simulink model "DFIG_and_Big_Generator"  (R2023a)
settings: Solver=ode45  StartTime=0.0  StopTime=10  RelTol=1e-2  EnableMultiTasking=on
PreLoadFcn:
  | assignin('base','Ts',[2e-6])
undefined symbols (not defined in the file): D1, Delta, DiscIntNeverNeededParam, find_system, Ion, level, Lithium, Ts
libraries: powerlib_extras x83, spsThreePhaseVIMeasurementLib x16, spsThreePhaseBreakerLib x16, simulink_extras x12, spsThreePhaseTransformerTwoWindingsLib x8, spsPLL3phLib x5, spsPowerPLLDrivenPositiveSequenceLib x5, spsUniversalBridgeLib x5, spsThreePhaseSeriesRLCLoadLib x5, spsThreePhaseSeriesRLCBranchLib x4, spsGroundLib x3, spsFundamentalPLLDrivenLib x2
(part 1 of 6)
settings Model: SimulationMode=accelerator  ExtModeTrigDuration=100  Creator=Administrator  LastModifiedBy=e36530cn
settings SolverCC: AlgebraicLoopSolver=TrustRegion
settings DataIOCC: LimitDataPoints=on  SaveFinalState=on  SaveFormat=Array  SignalLoggingSaveFormat=ModelDataLogs  SaveOutput=off  SaveState=on  ReturnWorkspaceOutputs=off  StateSaveName=tmp_raccel_xout
settings OptimizationCC: ExpressionDepthLimit=2147483647  EfficientMapNaN2IntZero=off  LifeSpan=inf
settings DebuggingCC: UnderspecifiedInitializationDetection=Classic  MergeDetectMultiDrivingBlocksExec=none  SolverPrmCheckMsg=warning  FcnCallInpInsideContextMsg=warning  UnconnectedInputMsg=warning  UnconnectedOutputMsg=warning  UnconnectedLineMsg=warning  StateNameClashWarn=warning  SFUnexpectedBacktrackingDiag=warning  SFNoUnconditionalDefaultTransitionDiag=warning  SFExecutionAtInitializationDiag=none  ArithmeticOperatorsInVariantConditions=warning
settings HardwareCC: ProdBitPerPointer=32  ProdBitPerSizeT=32  ProdBitPerPtrDiffT=32  ProdLargestAtomicFloat=None  ProdIntDivRoundTo=Undefined  ProdEndianess=Unspecified  ProdWordSize=32  ProdHWDeviceType=32-bit Generic  TargetBitPerPointer=64  TargetBitPerSizeT=64  TargetBitPerPtrDiffT=64  TargetLongLongMode=on  TargetIntDivRoundTo=Zero  TargetEndianess=LittleEndian  TargetWordSize=64  TargetHWDeviceType=MATLAB Host  ProdEqTarget=off
settings ModelReferenceCC: EnableRefExpFcnMdlSchedulingChecks=on  PropagateSignalLabelsOutOfModel=off
settings SFSimCC: SimUseLocalCustomCode=off  CustomCodeUndefinedFunction=UseInterfaceOnly
settings RTWCC: SystemTargetFile=raccel.tlc  TemplateMakefile=raccel_default_tmf  RTWVerbose=off  RTWUseLocalCustomCode=off  RTWUseSimCustomCode=on
settings CodeAppCC: GenerateComments=off  MaxIdLength=128  SimulinkBlockComments=off
settings RaccelTargetCC: ParMdlRefBuildCompliant=off  OptimizeReductions=off  ENABLE_SLEXEC_SSBRIDGE=0  RTWCAPISignals=off  RTWCAPIParams=off  RTWCAPIRootIO=off
settings ConfigComp: CovMetricSettings=dw  CovSaveCumulativeToWorkspaceVar=on  CovSaveSingleToWorkspaceVar=on  CovExternalEMLEnable=off
settings SimscapeCC: SimscapeNormalizeSystem=off

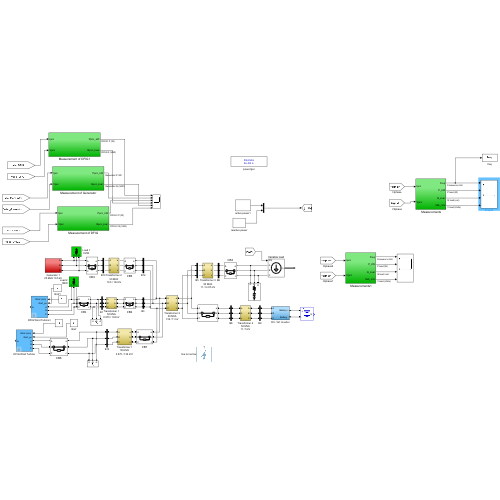
[thumbnail: Simulink's stored preview of the top-level diagram]
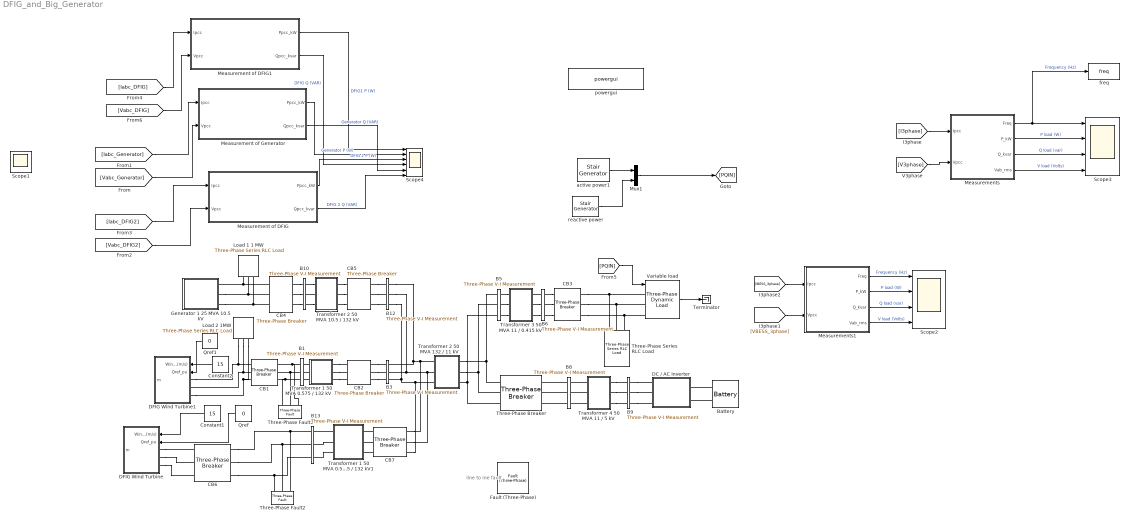
== system DFIG_and_Big_Generator ==
  note: line to ine fault
  " Measurements" : Subsystem
  " Measurements1" : Subsystem
  "B1 " : spsThreePhaseVIMeasurementLib/Three-Phase V-I Measurement  VoltageMeasurement=phase-to-ground  SetLabelV=on  LabelV=Vabc_DFIG  Vpu=off  VpuLL=off  CurrentMeasurement=yes  SetLabelI=on  LabelI=Iabc_DFIG  Ipu=off  Pbase=100e6  Vbase=735e3  OutputType=Complex  PhasorSimulation=off  PSBequivalent=0
  B10 : spsThreePhaseVIMeasurementLib/Three-Phase V-I Measurement  VoltageMeasurement=phase-to-ground  SetLabelV=on  LabelV=Vabc_Generator  Vpu=off  VpuLL=off  CurrentMeasurement=yes  SetLabelI=on  LabelI=Iabc_Generator  Ipu=off  Pbase=100e6  Vbase=735e3  OutputType=Complex  PhasorSimulation=off  PSBequivalent=0
  B12 : spsThreePhaseVIMeasurementLib/Three-Phase V-I Measurement  VoltageMeasurement=no  SetLabelV=on  LabelV=Vabc_B3  Vpu=off  VpuLL=off  CurrentMeasurement=no  SetLabelI=on  LabelI=Iabc_B2  Ipu=on  Pbase=100e6  Vbase=735e3  OutputType=Complex  PhasorSimulation=off  PSBequivalent=0
  B13 : spsThreePhaseVIMeasurementLib/Three-Phase V-I Measurement  VoltageMeasurement=phase-to-ground  SetLabelV=on  LabelV=Vabc_DFIG2  Vpu=off  VpuLL=off  CurrentMeasurement=yes  SetLabelI=on  LabelI=Iabc_DFIG2  Ipu=off  Pbase=100e6  Vbase=735e3  OutputType=Complex  PhasorSimulation=off  PSBequivalent=0
  "B3 " : spsThreePhaseVIMeasurementLib/Three-Phase V-I Measurement  VoltageMeasurement=no  SetLabelV=on  LabelV=Vabc_B3  Vpu=off  VpuLL=off  CurrentMeasurement=no  SetLabelI=on  LabelI=Iabc_B2  Ipu=on  Pbase=100e6  Vbase=735e3  OutputType=Complex  PhasorSimulation=off  PSBequivalent=0
  B5 : spsThreePhaseVIMeasurementLib/Three-Phase V-I Measurement  VoltageMeasurement=no  SetLabelV=on  LabelV=Vabc_B3  Vpu=off  VpuLL=off  CurrentMeasurement=no  SetLabelI=on  LabelI=Iabc_B2  Ipu=on  Pbase=100e6  Vbase=735e3  OutputType=Complex  PhasorSimulation=off  PSBequivalent=0
  B6 : spsThreePhaseVIMeasurementLib/Three-Phase V-I Measurement  VoltageMeasurement=phase-to-ground  SetLabelV=on  LabelV=V3phase  Vpu=off  VpuLL=off  CurrentMeasurement=yes  SetLabelI=on  LabelI=I3phase  Ipu=off  Pbase=100e6  Vbase=735e3  OutputType=Complex  PhasorSimulation=off  PSBequivalent=0
  B8 : spsThreePhaseVIMeasurementLib/Three-Phase V-I Measurement  VoltageMeasurement=no  SetLabelV=on  LabelV=Vabc_B3  Vpu=off  VpuLL=off  CurrentMeasurement=no  SetLabelI=on  LabelI=Iabc_B2  Ipu=on  Pbase=100e6  Vbase=735e3  OutputType=Complex  PhasorSimulation=off  PSBequivalent=0
  B9 : spsThreePhaseVIMeasurementLib/Three-Phase V-I Measurement  VoltageMeasurement=phase-to-ground  SetLabelV=on  LabelV=VBESS_3phase  Vpu=off  VpuLL=off  CurrentMeasurement=yes  SetLabelI=on  LabelI=IBESS_3phase  Ipu=off  Pbase=100e6  Vbase=735e3  OutputType=Complex  PhasorSimulation=off  PSBequivalent=0
  Battery : spsBatteryLib/Battery  BatType=Lithium-Ion  ShowTempParam=off  ThermalPreset=no  ShowAgeParam=off  NomV=5000  NomQ=13500  SOC=100  Batt_Tr=30  PresetModel=on  MaxQ=13500  MinV=3750  FullV=5819.9357  Dis_rate=5869.5652  R=0.0037037  Normal_OP=12208.6957  expZone="[5401.9293      663.26087]"  current=[2700 5400]  Units=Ampere-hour  Tci=20  NomT=25  T2=0  MaxQ2=2.208  FullV2=3.45  Normal_OP2=2.8  expZone2="[3.22        0.23]"  Rca=0.6  ti=1000  Dp=0  Neq0=0  Tsim=1e6  Ta1=25  Qeol=5.4*0.9  Reol=0.013333*1.2  Char_age=[2.3478, 3]  Dis_age=[2.3478, 10]  N1=1500  N2=10500  N3=1000  N4=1400  Ta2=45  N5=950
      settings: LibrarySourceBlock=electricdrivelib/Extra Sources/Battery
  CB{1..4} (4 alike) : spsThreePhaseBreakerLib/Three-Phase Breaker  InitialState=closed  SwitchA=off  SwitchB=off  SwitchC=off  SwitchTimes=[10]  External=off  BreakerResistance=1e-4  SnubberResistance=1e6  SnubberCapacitance=inf  Measurements=None
  CB5 : spsThreePhaseBreakerLib/Three-Phase Breaker  InitialState=closed  SwitchA=off  SwitchB=off  SwitchC=off  SwitchTimes=[1.360]  External=off  BreakerResistance=1e-4  SnubberResistance=1e6  SnubberCapacitance=inf  Measurements=None
  CB6 : spsThreePhaseBreakerLib/Three-Phase Breaker  InitialState=closed  SwitchA=off  SwitchB=off  SwitchC=off  SwitchTimes=[5,5.5]  External=off  BreakerResistance=1e-4  SnubberResistance=1e6  SnubberCapacitance=inf  Measurements=None
  CB7 : spsThreePhaseBreakerLib/Three-Phase Breaker  InitialState=closed  SwitchA=on  SwitchB=on  SwitchC=on  SwitchTimes=[5]  External=off  BreakerResistance=1e-4  SnubberResistance=1e6  SnubberCapacitance=inf  Measurements=None
  Constant1 : Constant  Value=15
  Constant2 : Constant  Value=15
  DC / AC Inverter : Subsystem
  DFIG Wind Turbine : Subsystem  LoadFcn=%find_system(gcs,'FollowLinks', 'on', 'LookUnderMasks', 'all');  mask(DFIG Wind Turbine){Nb_wt=8, ShowParameters=Turbine data for 1 wind turbine, nom=[1.5e6/.9 575 1975 50], sta=[ 0.023 0.18], rot=[ 0.016 0.16], Lm=2.9, mec=[0.685 0.01 3], init=[ -0.2,0   0,0,0   0,0,0 ], Imax_grid_conv=0.8, RL_grid=[ 0.3 0.003], Vdc_nom=1150, C_DClink1=10000e-6, C_var_filter1=120e3, Pmec1=1.5e6, wind_speed_CpMax=11, wind0=11, DisplayTurbChar=off, H_WT=4.32, Ksh=1.11, D_mutual=1.5, w_wt0=1.2, torque0=0.83, Kdc=[8   400], Kgrid_side_cur_reg=[0.83 5], Kspeed=[3 0.6], Krotor_side_cur_reg=[0.6 8], Ki_QV=[0.05 20], Kp_pitch=[150], Kcompensation=[3 30], PWM_freq_grid=2700, PWM_freq_rotor=1620, pitch_max=27, pitch_rate=10}
      mask prompts: Nb_wt "Number of wind turbines:"; ShowParameters "Display:"; nom "Nom. power, L-L volt. and freq. [Pn (VA), Vs_nom (Vrms), Vr_nom (Vrms), fn (Hz)]:"; sta "Stator [ Rs,Lls ] (p.u.):"; rot "Rotor [ Rr',Llr' ] (p.u.):"; Lm "Magnetizing inductance Lm (p.u.):"; mec "Inertia constant, friction factor, and pairs of poles [ H(s)  F(p.u.)  p ]:"; init "Initial conditions [s  th  ias  ibs  ics  phaseas phasebs phasecs]:"; Imax_grid_conv "Grid-side converter maximum current (pu of generator nominal current):"; RL_grid "Grid-side coupling inductor [ L, R] (p.u.):"; Vdc_nom "Nominal DC bus voltage (V):"; C_DClink1 "DC bus capacitor (F):"; C_var_filter1 "Line filter capacitor (Q=50) (var):"; Pmec1 "Nominal mechanical output power (W):"; wind_speed_CpMax "Wind speed at nominal speed and at Cp max (must be between 6 m/s and 30 m/s) (m/s):"; wind0 "Initial wind speed (m/s):"; DisplayTurbChar "Display wind turbine power characteristics:"; H_WT "Wind turbine inertia constant H (s):"; Ksh "Shaft spring constant refer to high-speed shaft (pu of nominal mechanical torque/rad):"; D_mutual "Shaft mutual damping (pu of nominal mechanical torque/pu dw):"; w_wt0 "Turbine initial speed (pu of nominal speed):"; torque0 "Initial output torque (pu of nominal mechanical torque):"; Kdc "DC bus voltage regulator gains [Kp Ki]:"; Kgrid_side_cur_reg "Grid-side converter current regulator gains [Kp Ki]:"; Kspeed "Speed regulator gains [Kp Ki]:"; Krotor_side_cur_reg "Rotor-side converter current regulator gains [Kp Ki]:"; Ki_QV "Q and V regulator gains [Ki_var Ki_volt]:"; Kp_pitch "Pitch controller gain [Kp]:"; Kcompensation "Pitch compensation gains [Kp Ki]:"; PWM_freq_grid "Frequency of the grid-side PWM carrier (Hz):"; PWM_freq_rotor "Frequency of the rotor-side PWM carrier (Hz):"; pitch_max "Maximum pitch angle (deg):"; pitch_rate "Maximum rate of change of pitch angle (deg/s):"
      mask help: This block implements a model of a variable speed pitch controlled wind turbine using a doubly-fed induction generator (DFIG).
      mask init:
      | %Generator data
      | Pnom=nom(1)*Nb_wt;
      | Vnom=nom(2);
      | Vnom_r=nom(3);
      | Fnom=nom(4);
      | Rs=sta(1);
      | Lls=sta(2);
      | Rr=rot(1);
      | Llr=rot(2);
      | H=mec(1);
      | F=mec(2);
      | p=mec(3);
      | 
      | % Converters data
      | L_RL=RL_grid(1);
      | R_RL=RL_grid(2);
      | Q_filter=50;
      | C_DClink=C_DClink1*Nb_wt;
      | C_var_filter=C_var_filter1*Nb_wt;
      | 
      | % Controller data
      | Freq_filter=1000*10;   %Hz
      | Zeta_filter=0.707;
      | Mod_index_max_grid=1.1;   %Maximum value of modulation index for grid-side converter
      | Mod_index_max_rotor=2;   %Maximum value of modulation index for rotor-side converter
      | Lim_grid_side_cur_reg=1.1; %Limit for grid-side PI current regulator (pu)
      | Lim_rotor_side_cur_reg=0.1; %Limit for rotor-side PI current regulator (pu)
      | Min_var_reg=0.9; %Minimum output value for integral var regulator (pu)
      | Max_var_reg=1.1; %Maximum output value for integral var regulator (pu)
      | Max_speed_reg=1; %Maximum output value for PI speed regulator (pu)
      | Kp_dc=Kdc(1);
      | Ki_dc=Kdc(2);
      | Kp_grid_side_cur_reg=Kgrid_side_cur_reg(1);
      | Ki_grid_side_cur_reg=Kgrid_side_cur_reg(2);
      | Kp_speed=Kspeed(1);
      | Ki_speed=Kspeed(2);
      | Kp_compensation=Kcompensation(1);
      | Ki_compensation=Kcompensation(2);
      | Kp_rotor_side_cur_reg=Krotor_side_cur_reg(1);
      | Ki_rotor_side_cur_reg=Krotor_side_cur_reg(2);
      | Ki_var=Ki_QV(1);
      | Ki_volt=Ki_QV(2);
      | Iq_ref_limit_time_constant=0.3; %(s)
      | T_speed=5;      %s
      | Min_mag_flux=0.5;   %(pu)
      | Max_Idr_ref=0.9;    %(pu)
      | Speed_max=1.2;  %(pu)
      | Speed_min=0.7;  %(pu)
      | Pitch_time_constant=0.01;    %(s)
      | 
      | 
      | % Turbine data
      | Pmec=Pmec1*Nb_wt;
      | c1 = 0.6450;
      | c2 = 116;
      | c3 = .4;
      | c4 = 5;
      | c5 = 21;
      | c6 = .00912;  % Set Pmin in stall condition (does not vary with wind_speed_Pmax)
      | c7 = .08;
      | c8 = .035;
      | theta=0;
      | CpMax=.5;
      | lambda_CpMax=9.9495;
      | 
      | c1_c8=[c1 c2 c3 c4 c5 c6 c7 c8];
      |   
      | 
      | %   Cp = c1*(c6*lambda + (-c4 - c3*(2.5 + theta) + c2*(1/(lambda + ...
      | %   c7*(2.5 + theta)) - c8/(1 + (2.5 + theta)^3)))/exp(c5*(1/(lambda + ...
      | %   c7*(2.5 + theta)) - c8/(1 + (2.5 + theta)^3))))
      | 
      | 
      |         %%%%%%%%%%%%%%%%%%%%%%%%%%%%%%%%%%%%%%%%%%%%%%%%%%%%%%%%%%%%%%%%%%%%%%%%%%%
      |         % Operation at Cp max
      |         %%%%%%%%%%%%%%%%%%%%%%%%%%%%%%%%%%%%%%%%%%%%%%%%%%%%%%%%%%%%%%%%%%%%%%%%%%%
      |         
      |         rated_omegar=1.2;
      |         omegar = rated_omegar;
      |         
      |         % Enforce boundaries on wind speed
      |         % A warning could be displayed
      |         if wind_speed_CpMax < 6
      |             wind_speed_CpMax=6;
      |             disp('Warning: Wind speed at nominal speed and at Cp max has been set to 6 m/s')
      |         end
      |         if wind_speed_CpMax > 30
      |             wind_speed_CpMax=30;
      |             disp('Warning: Wind speed at nominal speed and at Cp max has been set to 30 m/s')
      |         end
      | 
      |         K1=lambda_CpMax/omegar*wind_speed_CpMax;
      |         
      |         % Calculation of K2 needed to get P equal to the requested value at
      |         % Cp max for the requested wind speed
      |         
      |         Prated=Pmec1*Nb_wt;
      |         P_rated_omegar_theta_zero=0.75;
      |         
      |         K2 = P_rated_omegar_theta_zero*Prated/(wind_speed_CpMax^3*CpMax);
      |         
      |         K1_K2=[K1 K2];
      |         
      |         %%%%%%%%%%%%%%%%%%%%%%%%%%%%%%%%%%%%%%%%%%%%%%%%%%%%%%%%%%%%%%%%%%%%%%%%%%%
      |         % End of calculation for operation at Cp max
      |         %%%%%%%%%%%%%%%%%%%%%%%%%%%%%%%%%%%%%%%%%%%%%%%%%%%%%%%%%%%%%%%%%%%%%%%%%%%
      |         
      | 
      | %%%%%%%%%%%%%%%%%%%%%%%%%%%%%%%%%%%%%%%%%%%%%%%%%%%%%%%%%%%%%%%%%%%%%%%%%%%
      | % Plot turbine characteristics
      | %%%%%%%%%%%%%%%%%%%%%%%%%%%%%%%%%%%%%%%%%%%%%%%%%%%%%%%%%%%%%%%%%%%%%%%%%%% 
      | 
      | DisplayTurbChar=get_param(gcb,'DisplayTurbChar');
      | if strcmp(DisplayTurbChar,'on')
      |     vect_theta = 0:2:30;
      |     
      |     vect_lambda = 1:0.2:30;
      |     
      |     clear Cp;
      |     
      |     for i=1:length(vect_theta)
      |      for j=1:length(vect_lambda)
      |                 Cp(i,j) = c1*(c6*vect_lambda(j) + (-c4 - c3*(2.5 + vect_theta(i)) + c2*(1/(vect_lambda(j) + ...
      |                 c7*(2.5 + vect_theta(i))) - c8/(1 + (2.5 + vect_theta(i))^3)))/exp(c5*(1/(vect_lambda(j) + ...
      |                 c7*(2.5 + vect_theta(i))) - c8/(1 + (2.5 + vect_theta(i))^3))));
      |      end
      |     end
      | 
      |     figure(1);
      |     clf;
      |     hold on;
      | 
      |     plot(vect_lambda, Cp);
      |     axis([0, 25, 0, .6]);
      |     title('Wind Turbine Cp Characteristic (pitch angle increases by step of 2 deg.)');
      |     ylabel('Cp');
      |     set(gca,'ytick',[0 .1 .2 .3 .4 .5 .6]);
      |     xlabel('Lambda');
      |     grid on;
      |     text(10.1,0.51,'Pitch angle 0 degree');
      | 
      |     hold off
      |     
      |     % Plot of the wind turbine mechanical power output (pu) lambda and Cp
      |     % characteristics against wind speed (m/s) for a range of theta.
      |     
      |     wind_speed_range = [1,.2,30];
      |     vect_wind_speed = 1:0.2:30;
      |     
      |     clear lambda;
      |     clear Cp;
      |     clear P;
      | 
      |     for i=1:length(vect_theta)
      |         for j=1:length(vect_wind_speed)
      |             lambda(i,j) = K1*omegar/vect_wind_speed(j);
      |             Cp(i,j) = c1*(c6*lambda(i,j) + (-c4 - c3*(2.5 + vect_theta(i)) + c2*(1/(lambda(i,j) + ...
      |             c7*(2.5 + vect_theta(i))) - c8/(1 + (2.5 + vect_theta(i))^3)))/exp(c5*(1/(lambda(i,j) + ...
      |             c7*(2.5 + vect_theta(i))) - c8/(1 + (2.5 + vect_theta(i))^3))));
      |             P(i,j) = K2/Prated*vect_wind_speed(j)^3*Cp(i,j);
      |         end
      |     end
      |     
      |     
      |     figure(2);
      |     clf;
      |     hold on
      |     
      |     subplot(3,1,1);
      |     plot(vect_wind_speed, P);
      |     axis([0, 35, 0, 1.5]);
      |     title('Wind Turbine Characteristics (w = 1.2 pu, pitch angle increases by step of 2 deg.)');
      |     ylabel('P (pu)');
      |     set(gca,'ytick',0:.5:4);
      |     grid on;
      |     
      |     subplot(3,1,2);
      |     plot(vect_wind_speed, lambda);
      |     axis([0, 35, 0, 20]);
      |     ylabel('Lambda');
      |     grid on;
      |     
      |     subplot(3,1,3)
      |     plot(vect_wind_speed, Cp);
      |     axis([0, 35, 0, .6]);
      |     xlabel('Wind Speed (m/s)');
      |     ylabel('Cp');
      |     set(gca,'ytick',[0 .1 .2 .3 .4 .5 .6]);
      |     grid on;
      | 
      |     hold off
      |     set_param(gcb,'DisplayTurbChar','off')
      |     
      | end
      mask TypeOptions ShowParameters: Generator data for 1 wind turbine | Converters data for 1 wind turbine | Turbine data for 1 wind turbine | Drive train data for 1 wind turbine | Control parameters for 1 wind turbine
      mask Callback ShowParameters:
      | BlockName=getfullname(gcb);
      | %
      | Param_Show=get_param(BlockName,'ShowParameters');
      | Param_DisplayTurbChar=get_param(BlockName,'DisplayTurbChar');
      | 
      | p_mask{3}='off';p_mask{4}='off';p_mask{5}='off';
      | p_mask{6}='off';p_mask{7}='off';p_mask{8}='off';p_mask{9}='off';
      | p_mask{10}='off';p_mask{11}='off';p_mask{12}='off';p_mask{13}='off';
      | p_mask{14}='off';p_mask{15}='off';p_mask{16}='off';p_mask{17}='off';
      | p_mask{18}='off';p_mask{19}='off';p_mask{20}='off';p_mask{21}='off';
      | p_mask{22}='off';p_mask{23}='off';p_mask{24}='off';p_mask{25}='off';
      | p_mask{26}='off';p_mask{27}='off';p_mask{28}='off';p_mask{29}='off';
      | p_mask{30}='off';p_mask{31}='off';p_mask{32}='off';p_mask{33}='off';
      | 
      | 
      | switch Param_Show
      | 	case 'Generator data for 1 wind turbine'
      | 		p_mask{3}='on';p_mask{4}='on';p_mask{5}='on'; p_mask{6}='on';
      |         p_mask{7}='on'; p_mask{8}='on';
      |     case 'Converters data for 1 wind turbine'
      | 		p_mask{9}='on';p_mask{10}='on';p_mask{11}='on';p_mask{12}='on';
      |         p_mask{13}='on';
      | 	case 'Turbine data for 1 wind turbine'
      |         p_mask{14}='on';p_mask{15}='on';p_mask{16}='on';p_mask{17}='on';
      |     case 'Drive train data for 1 wind turbine'
      |         p_mask{18}='on';p_mask{19}='on';p_mask{20}='on';p_mask{21}='on';
      |         p_mask{22}='on';
      |     case 'Control parameters for 1 wind turbine'
      |         p_mask{23}='on';p_mask{24}='on';p_mask{25}='on';
      |         p_mask{26}='on';p_mask{27}='on';p_mask{28}='on';p_mask{29}='on';
      |         p_mask{30}='on'; p_mask{31}='on';p_mask{32}='on'; p_mask{33}='on';
      | end
      | 
      | ParVisible={'on','on',p_mask{3},p_mask{4},p_mask{5},p_mask{6},p_mask{7},...
      |     p_mask{8},p_mask{9},p_mask{10},p_mask{11},p_mask{12},p_mask{13},...
      |     p_mask{14},p_mask{15},p_mask{16},p_mask{17},p_mask{18},p_mask{19},...
      |     p_mask{20},p_mask{21},p_mask{22},p_mask{23},p_mask{24},p_mask{25},...
      |     p_mask{26},p_mask{27},p_mask{28},p_mask{29},p_mask{30},p_mask{31},...
      |     p_mask{32},p_mask{33}};
      | %
      | set_param(BlockName,'MaskVisibilities',ParVisible);
      | set_param(BlockName,'DisplayTurbChar',Param_DisplayTurbChar);
  DFIG Wind Turbine1 : Subsystem  LoadFcn=%find_system(gcs,'FollowLinks', 'on', 'LookUnderMasks', 'all');  mask(DFIG Wind Turbine){Nb_wt=9, ShowParameters=Turbine data for 1 wind turbine, nom=[1.5e6/.9 575 1975 50], sta=[ 0.023 0.18], rot=[ 0.016 0.16], Lm=2.9, mec=[0.685 0.01 3], init=[ -0.2,0   0,0,0   0,0,0 ], Imax_grid_conv=0.8, RL_grid=[ 0.3 0.003], Vdc_nom=1150, C_DClink1=10000e-6, C_var_filter1=120e3, Pmec1=1.5e6, wind_speed_CpMax=11, wind0=11, DisplayTurbChar=off, H_WT=4.32, Ksh=1.11, D_mutual=1.5, w_wt0=1.2, torque0=0.83, Kdc=[8   400], Kgrid_side_cur_reg=[0.83 5], Kspeed=[3 0.6], Krotor_side_cur_reg=[0.6 8], Ki_QV=[0.05 20], Kp_pitch=[150], Kcompensation=[3 30], PWM_freq_grid=2700, PWM_freq_rotor=1620, pitch_max=27, pitch_rate=10}
      mask prompts: Nb_wt "Number of wind turbines:"; ShowParameters "Display:"; nom "Nom. power, L-L volt. and freq. [Pn (VA), Vs_nom (Vrms), Vr_nom (Vrms), fn (Hz)]:"; sta "Stator [ Rs,Lls ] (p.u.):"; rot "Rotor [ Rr',Llr' ] (p.u.):"; Lm "Magnetizing inductance Lm (p.u.):"; mec "Inertia constant, friction factor, and pairs of poles [ H(s)  F(p.u.)  p ]:"; init "Initial conditions [s  th  ias  ibs  ics  phaseas phasebs phasecs]:"; Imax_grid_conv "Grid-side converter maximum current (pu of generator nominal current):"; RL_grid "Grid-side coupling inductor [ L, R] (p.u.):"; Vdc_nom "Nominal DC bus voltage (V):"; C_DClink1 "DC bus capacitor (F):"; C_var_filter1 "Line filter capacitor (Q=50) (var):"; Pmec1 "Nominal mechanical output power (W):"; wind_speed_CpMax "Wind speed at nominal speed and at Cp max (must be between 6 m/s and 30 m/s) (m/s):"; wind0 "Initial wind speed (m/s):"; DisplayTurbChar "Display wind turbine power characteristics:"; H_WT "Wind turbine inertia constant H (s):"; Ksh "Shaft spring constant refer to high-speed shaft (pu of nominal mechanical torque/rad):"; D_mutual "Shaft mutual damping (pu of nominal mechanical torque/pu dw):"; w_wt0 "Turbine initial speed (pu of nominal speed):"; torque0 "Initial output torque (pu of nominal mechanical torque):"; Kdc "DC bus voltage regulator gains [Kp Ki]:"; Kgrid_side_cur_reg "Grid-side converter current regulator gains [Kp Ki]:"; Kspeed "Speed regulator gains [Kp Ki]:"; Krotor_side_cur_reg "Rotor-side converter current regulator gains [Kp Ki]:"; Ki_QV "Q and V regulator gains [Ki_var Ki_volt]:"; Kp_pitch "Pitch controller gain [Kp]:"; Kcompensation "Pitch compensation gains [Kp Ki]:"; PWM_freq_grid "Frequency of the grid-side PWM carrier (Hz):"; PWM_freq_rotor "Frequency of the rotor-side PWM carrier (Hz):"; pitch_max "Maximum pitch angle (deg):"; pitch_rate "Maximum rate of change of pitch angle (deg/s):"
      mask help: This block implements a model of a variable speed pitch controlled wind turbine using a doubly-fed induction generator (DFIG).
      mask init: same as DFIG_and_Big_Generator/DFIG Wind Turbine
      mask TypeOptions ShowParameters: Generator data for 1 wind turbine | Converters data for 1 wind turbine | Turbine data for 1 wind turbine | Drive train data for 1 wind turbine | Control parameters for 1 wind turbine
      mask Callback ShowParameters:
      | BlockName=getfullname(gcb);
      | %
      | Param_Show=get_param(BlockName,'ShowParameters');
      | Param_DisplayTurbChar=get_param(BlockName,'DisplayTurbChar');
      | 
      | p_mask{3}='off';p_mask{4}='off';p_mask{5}='off';
      | p_mask{6}='off';p_mask{7}='off';p_mask{8}='off';p_mask{9}='off';
      | p_mask{10}='off';p_mask{11}='off';p_mask{12}='off';p_mask{13}='off';
      | p_mask{14}='off';p_mask{15}='off';p_mask{16}='off';p_mask{17}='off';
      | p_mask{18}='off';p_mask{19}='off';p_mask{20}='off';p_mask{21}='off';
      | p_mask{22}='off';p_mask{23}='off';p_mask{24}='off';p_mask{25}='off';
      | p_mask{26}='off';p_mask{27}='off';p_mask{28}='off';p_mask{29}='off';
      | p_mask{30}='off';p_mask{31}='off';p_mask{32}='off';p_mask{33}='off';
      | 
      | 
      | switch Param_Show
      | 	case 'Generator data for 1 wind turbine'
      | 		p_mask{3}='on';p_mask{4}='on';p_mask{5}='on'; p_mask{6}='on';
      |         p_mask{7}='on'; p_mask{8}='on';
      |     case 'Converters data for 1 wind turbine'
      | 		p_mask{9}='on';p_mask{10}='on';p_mask{11}='on';p_mask{12}='on';
      |         p_mask{13}='on';
      | 	case 'Turbine data for 1 wind turbine'
      |         p_mask{14}='on';p_mask{15}='on';p_mask{16}='on';p_mask{17}='on';
      |     case 'Drive train data for 1 wind turbine'
      |         p_mask{18}='on';p_mask{19}='on';p_mask{20}='on';p_mask{21}='on';
      |         p_mask{22}='on';
      |     case 'Control parameters for 1 wind turbine'
      |         p_mask{23}='on';p_mask{24}='on';p_mask{25}='on';
      |         p_mask{26}='on';p_mask{27}='on';p_mask{28}='on';p_mask{29}='on';
      |         p_mask{30}='on'; p_mask{31}='on';p_mask{32}='on'; p_mask{33}='on';
      | end
      | 
      | ParVisible={'on','on',p_mask{3},p_mask{4},p_mask{5},p_mask{6},p_mask{7},...
      |     p_mask{8},p_mask{9},p_mask{10},p_mask{11},p_mask{12},p_mask{13},...
      |     p_mask{14},p_mask{15},p_mask{16},p_mask{17},p_mask{18},p_mask{19},...
      |     p_mask{20},p_mask{21},p_mask{22},p_mask{23},p_mask{24},p_mask{25},...
      |     p_mask{26},p_mask{27},p_mask{28},p_mask{29},p_mask{30},p_mask{31},...
      |     p_mask{32},p_mask{33}};
      | %
      | set_param(BlockName,'MaskVisibilities',ParVisible);
      | set_param(BlockName,'DisplayTurbChar',Param_DisplayTurbChar);
  Fault (Three-Phase) : ee_lib/Utilities/Fault (Three-Phase)  fault_type_option=0  R_pn_fault=1e-3 Ohm  R_ng_fault=1e-3 Ohm  exposemeasurement=ee.enum.exposemeasurement.hidden  enable_external_fault=ee.enum.external_fault.hidden  fault_threshold=0.5  fault_condition=1  fault_resettable=0  enable_temporal_fault=0  fault_start_time=1 s  fault_duration=0.1 s  G_parasitic=1e-6 1/Ohm
      settings: InternalSimscapePortConfiguration="{\"Bottom\":[],\"Left\":[{\"id\":\"N\",\"label\":\"~\",\"type\":\"foundation.electrical.three_phase\"}],\"Right\":[],\"Top\":[]}"
  Generator 1 25 MVA 10.5 kV : Subsystem
  Load 1 1 MW : spsThreePhaseSeriesRLCLoadLib/Three-Phase Series RLC Load  LConnTagsString=A|B|C  Configuration=Y (grounded)  NominalVoltage=10.5e3  Vabc=[1e3 1e3 1e3]  Vabcp=[1e3 1e3 1e3]  NominalFrequency=50  UnbalancedPower=off  ActivePower=1e6  InductivePower=0  CapacitivePower=0  Pabc=[10e3 9e3 11e3]  QLabc=[100 90 110]  QCabc=[100 90 110]  Pabcp=[10e3 9e3 11e3]  QLabcp=[100 90 110]  QCabcp=[100 90 110]  Measurements=None  LoadType=constant Z
  Load 2 1MW : spsThreePhaseSeriesRLCLoadLib/Three-Phase Series RLC Load  LConnTagsString=A|B|C  Configuration=Y (grounded)  NominalVoltage=575  Vabc=[1e3 1e3 1e3]  Vabcp=[1e3 1e3 1e3]  NominalFrequency=50  UnbalancedPower=off  ActivePower=1e6  InductivePower=0  CapacitivePower=0  Pabc=[10e3 9e3 11e3]  QLabc=[100 90 110]  QCabc=[100 90 110]  Pabcp=[10e3 9e3 11e3]  QLabcp=[100 90 110]  QCabcp=[100 90 110]  Measurements=None  LoadType=constant Z
  Measurement of DFIG : Subsystem
  Measurement of DFIG1 : Subsystem
  Measurement of Generator : Subsystem
  Mux1 : Mux  Inputs=2
  Qref : Constant  Value=0
  Qref1 : Constant  Value=0
  Scope2 : Scope  NumInputPorts=4
  Scope3 : Scope  NumInputPorts=4
  Scope4 : Scope  NumInputPorts=6
  Terminator : Terminator
  Three-Phase Series RLC Load : spsThreePhaseSeriesRLCLoadLib/Three-Phase Series RLC Load  LConnTagsString=A|B|C  Configuration=Y (grounded)  NominalVoltage=415  Vabc=[1e3 1e3 1e3]  Vabcp=[1e3 1e3 1e3]  NominalFrequency=50  UnbalancedPower=off  ActivePower=15E6  InductivePower=0  CapacitivePower=27E6  Pabc=[10e3 9e3 11e3]  QLabc=[100 90 110]  QCabc=[100 90 110]  Pabcp=[10e3 9e3 11e3]  QLabcp=[100 90 110]  QCabcp=[100 90 110]  Measurements=None  LoadType=constant Z
  Three-Phase Breaker : spsThreePhaseBreakerLib/Three-Phase Breaker  InitialState=closed  SwitchA=off  SwitchB=off  SwitchC=off  SwitchTimes="[1/60  5/60]"  External=off  BreakerResistance=0.01  SnubberResistance=1e6  SnubberCapacitance=inf  Measurements=None
  Three-Phase Fault1 : spsThreePhaseFaultLib/Three-Phase Fault  InitialStates=0  FaultA=on  FaultB=off  FaultC=off  GroundFault=off  SwitchTimes=[ 5]  External=off  SwitchStatus=NaN  FaultResistance=0.001  GroundResistance=0.01  SnubberResistance=1e6  SnubberCapacitance=inf  Measurements=None
  Three-Phase Fault2 : spsThreePhaseFaultLib/Three-Phase Fault  InitialStates=0  FaultA=off  FaultB=off  FaultC=off  GroundFault=off  SwitchTimes=[5]  External=off  SwitchStatus=NaN  FaultResistance=0.001  GroundResistance=0.01  SnubberResistance=1e6  SnubberCapacitance=inf  Measurements=None
  Transformer 1 50 MVA 0.575 / 132 kV : Subsystem
  Transformer 1 50 MVA 0.575 / 132 kV1 : Subsystem
  Transformer 2 50 MVA 10.5 / 132 kV : Subsystem
  Transformer 2 50 MVA 132 / 11 kV : Subsystem
  Transformer 3 50 MVA 11 / 0.415 kV : Subsystem
  Transformer 4 50 MVA 11 / 5 kV : Subsystem
  Variable load : spsThreePhaseDynamicLoadLib/Three-Phase Dynamic Load  NominalVoltage=[ 415 50 ]  ActiveReactivePowers=[15e6 0E6]  PositiveSequence=[1 0]  ExternalControl=on  NpNq=[1.3 2]  TimeConstants="[0  0  0  0]"  MinimumVoltage=0.7  Tfilter=1e-4  LoadFlowParameters=[4,0,0,0,0]
  active power1 : spsStairGeneratorLib/Stair Generator  t=[0]  e=[15E6]  Ts=0
  freq : ToWorkspace  VariableName=freq  SaveFormat=Structure With Time  SampleTime=-1
  powergui : sps_lib/powergui  Priority=1  SimulationMode=Discrete  SampleTime=Ts  frequency=60  Iterations=50  frequencyindice=0  Pbase=100e6  ErrMax=1e-4  UnitsV=kV  UnitsW=MW  buscounter=0  FunctionMessages=off  echomessages=off  EnableUseOfTLC=off  CurrentSourceSwitches=off  DisableSnubberDevices=off  DisableRonSwitches=off  DisableVfSwitches=off  DisplayEquations=off  AutomaticDiscreteSolvers=off  SolverType=Tustin  Interpol=off  ExternalGateDelay=off  methode=off  Ts=10  x0status=blocks  SPID=off  SwTol=0  HookPort=off  NonlinearTolerance=1e-4  nMaxIteration=100  ContinueOnMaxIteration=off  RestoreLinks=warning  ResistiveCurrentMeasurement=off  Frange=[0:2:500]  Ylog=off  Xlog=on  ShowGrid=off  save=off  variable=ZData  structure=psbbridges_str  ZoomFFT=off  StartTime=0.0  cycles=1  DisplayStyle=1  fundamental=50  FreqAxis=off  MaxFrequency=100  frequencyindicesteady=1  RmsSteady=2  display=off
  reactive power : spsStairGeneratorLib/Stair Generator  t=[0]  e=[0]  Ts=0
  Scope1 : Scope
  wires:
  [V3phase] -> " Measurements"/2(Vpcc)
  " Measurements"/1(Freq) -> freq/1, Scope3/1  "Frequency (Hz)"
  [I3phase] -> " Measurements"/1(Ipcc)
  " Measurements"/3(Q_kvar) -> Scope3/3  "Q load (var)"
  " Measurements"/2(P_kW) -> Scope3/2  "P load (W)"
  " Measurements"/4(Vab_rms) -> Scope3/4  "V load (Volts)"
  Measurement of DFIG/1(Ppcc_kW) -> Scope4/3  "DFIG 2 P (W)"
  Measurement of DFIG/2(Qpcc_kvar) -> Scope4/6  "DFIG 2 Q (VAR)"
  [Vabc_Generator] -> Measurement of Generator/2(Vpcc)
  [Iabc_Generator] -> Measurement of Generator/1(Ipcc)
  [Vabc_DFIG2] -> Measurement of DFIG/2(Vpcc)
  [Iabc_DFIG2] -> Measurement of DFIG/1(Ipcc)
  Qref/1 -> DFIG Wind Turbine/2(Qref_pu)
  Constant1/1 -> DFIG Wind Turbine/1("Wind (m/s) ")
  Qref1/1 -> DFIG Wind Turbine1/2(Qref_pu)
  Constant2/1 -> DFIG Wind Turbine1/1("Wind (m/s) ")
  [Iabc_DFIG] -> Measurement of DFIG1/1(Ipcc)
  [Vabc_DFIG] -> Measurement of DFIG1/2(Vpcc)
  Measurement of DFIG1/2(Qpcc_kvar) -> Scope4/4  "DFIG Q (VAR)"
  Measurement of DFIG1/1(Ppcc_kW) -> Scope4/1  "DFIG1 P (W)"
  Variable load/1 -> Terminator/1
  Mux1/1 -> [PQIN]
  reactive power/1 -> Mux1/2
  active power1/1 -> Mux1/1
  Measurement of Generator/1(Ppcc_kW) -> Scope4/2  "Generator P (W)"
  Measurement of Generator/2(Qpcc_kvar) -> Scope4/5  "Generator Q (VAR)"
  [PQIN] -> Variable load/1
  [IBESS_3phase] -> " Measurements1"/1(Ipcc)
  [VBESS_3phase] -> " Measurements1"/2(Vpcc)
  " Measurements1"/2(P_kW) -> Scope2/2  "P load (W)"
  " Measurements1"/3(Q_kvar) -> Scope2/3  "Q load (var)"
  " Measurements1"/4(Vab_rms) -> Scope2/4  "V load (Volts)"
  " Measurements1"/1(Freq) -> Scope2/1  "Frequency (Hz)"
  connections:
  CB3/RConn1 -- Three-Phase Series RLC Load/LConn1 -- Variable load/LConn1
  CB3/RConn3 -- Three-Phase Series RLC Load/LConn3 -- Variable load/LConn3
  Transformer 2 50 MVA 132 / 11 kV/LConn1 -- CB7/RConn1 -- B12/RConn1 -- "B3 "/RConn1
  Transformer 2 50 MVA 132 / 11 kV/LConn2 -- CB7/RConn2 -- B12/RConn2 -- "B3 "/RConn2
  Transformer 2 50 MVA 132 / 11 kV/LConn3 -- CB7/RConn3 -- B12/RConn3 -- "B3 "/RConn3
  B6/RConn2 -- CB3/LConn2
  "B1 "/LConn1 -- CB1/RConn1 -- Three-Phase Fault1/LConn1
  Transformer 1 50 MVA 0.575 / 132 kV/LConn3 -- "B1 "/RConn3
  Transformer 1 50 MVA 0.575 / 132 kV/LConn2 -- "B1 "/RConn2
  Transformer 2 50 MVA 132 / 11 kV/RConn2 -- B5/LConn2 -- Three-Phase Breaker/LConn2
  Transformer 2 50 MVA 132 / 11 kV/RConn1 -- B5/LConn1 -- Three-Phase Breaker/LConn1
  B5/RConn1 -- Transformer 3 50 MVA 11 / 0.415 kV/RConn1
  B5/RConn2 -- Transformer 3 50 MVA 11 / 0.415 kV/RConn2
  B5/RConn3 -- Transformer 3 50 MVA 11 / 0.415 kV/RConn3
  Transformer 3 50 MVA 11 / 0.415 kV/LConn2 -- B6/LConn2
  Transformer 3 50 MVA 11 / 0.415 kV/LConn3 -- B6/LConn3
  B6/RConn1 -- CB3/LConn1
  B6/RConn3 -- CB3/LConn3
  CB3/RConn2 -- Three-Phase Series RLC Load/LConn2 -- Variable load/LConn2
  CB2/RConn1 -- "B3 "/LConn1
  CB2/RConn2 -- "B3 "/LConn2
  CB2/RConn3 -- "B3 "/LConn3
  "B1 "/LConn2 -- CB1/RConn2 -- Three-Phase Fault1/LConn2
  "B1 "/LConn3 -- Three-Phase Fault1/LConn3 -- CB1/RConn3
  B6/LConn1 -- Transformer 3 50 MVA 11 / 0.415 kV/LConn1
  Transformer 4 50 MVA 11 / 5 kV/RConn2 -- B8/RConn2
  Transformer 4 50 MVA 11 / 5 kV/RConn1 -- B8/RConn1
  Battery/LConn1 -- DC / AC Inverter/LConn1
  Transformer 4 50 MVA 11 / 5 kV/LConn2 -- B9/LConn2
  Battery/LConn2 -- DC / AC Inverter/LConn2
  Transformer 4 50 MVA 11 / 5 kV/LConn3 -- B9/LConn3
  Transformer 4 50 MVA 11 / 5 kV/RConn3 -- B8/RConn3
  Transformer 4 50 MVA 11 / 5 kV/LConn1 -- B9/LConn1
  CB4/RConn1 -- B10/LConn1
  CB5/RConn3 -- B12/LConn3
  CB5/RConn1 -- B12/LConn1
  B10/RConn3 -- Transformer 2 50 MVA 10.5 / 132 kV/LConn3
  CB5/RConn2 -- B12/LConn2
  B10/RConn1 -- Transformer 2 50 MVA 10.5 / 132 kV/LConn1
  CB4/RConn2 -- B10/LConn2
  CB4/RConn3 -- B10/LConn3
  B9/RConn2 -- DC / AC Inverter/RConn2
  B9/RConn1 -- DC / AC Inverter/RConn1
  B9/RConn3 -- DC / AC Inverter/RConn3
  Load 1 1 MW/LConn1 -- Generator 1 25 MVA 10.5 kV/RConn1 -- CB4/LConn1
  Generator 1 25 MVA 10.5 kV/RConn2 -- Load 1 1 MW/LConn2 -- CB4/LConn2
  Generator 1 25 MVA 10.5 kV/RConn3 -- CB4/LConn3 -- Load 1 1 MW/LConn3
  B8/LConn1 -- Three-Phase Breaker/RConn1
  B8/LConn2 -- Three-Phase Breaker/RConn2
  B8/LConn3 -- Three-Phase Breaker/RConn3
  Transformer 2 50 MVA 132 / 11 kV/RConn3 -- B5/LConn3 -- Three-Phase Breaker/LConn3
  Load 2 1MW/LConn2 -- DFIG Wind Turbine1/LConn2 -- CB1/LConn2
  Load 2 1MW/LConn3 -- DFIG Wind Turbine1/LConn3 -- CB1/LConn3
  DFIG Wind Turbine/LConn1 -- CB6/LConn1
  DFIG Wind Turbine/LConn2 -- CB6/LConn2
  DFIG Wind Turbine/LConn3 -- CB6/LConn3
  Load 2 1MW/LConn1 -- CB1/LConn1 -- DFIG Wind Turbine1/LConn1
  Transformer 2 50 MVA 10.5 / 132 kV/LConn2 -- B10/RConn2
  Transformer 2 50 MVA 10.5 / 132 kV/RConn1 -- CB5/LConn1
  Transformer 2 50 MVA 10.5 / 132 kV/RConn2 -- CB5/LConn2
  Transformer 2 50 MVA 10.5 / 132 kV/RConn3 -- CB5/LConn3
  Transformer 1 50 MVA 0.575 / 132 kV/RConn1 -- CB2/LConn1
  Transformer 1 50 MVA 0.575 / 132 kV/RConn2 -- CB2/LConn2
  Transformer 1 50 MVA 0.575 / 132 kV/RConn3 -- CB2/LConn3
  "B1 "/RConn1 -- Transformer 1 50 MVA 0.575 / 132 kV/LConn1
  CB6/RConn3 -- Three-Phase Fault2/LConn3 -- B13/LConn3
  CB6/RConn2 -- Three-Phase Fault2/LConn2 -- B13/LConn2
  CB6/RConn1 -- B13/LConn1 -- Three-Phase Fault2/LConn1
  Transformer 1 50 MVA 0.575 / 132 kV1/LConn1 -- B13/RConn1
  Transformer 1 50 MVA 0.575 / 132 kV1/LConn2 -- B13/RConn2
  Transformer 1 50 MVA 0.575 / 132 kV1/LConn3 -- B13/RConn3
  CB7/LConn1 -- Transformer 1 50 MVA 0.575 / 132 kV1/RConn1
  CB7/LConn2 -- Transformer 1 50 MVA 0.575 / 132 kV1/RConn2
  CB7/LConn3 -- Transformer 1 50 MVA 0.575 / 132 kV1/RConn3

== system DFIG_and_Big_Generator/ Measurements ==
  Ipcc : Inport
  Vpcc : Inport  Port=2
  Add1 : Sum  Inputs=+-
  Demux1 : Demux  Outputs=3
  Fundamental (PLL-Driven) : spsFundamentalPLLDrivenLib/Fundamental (PLL-Driven)  Finit=50  Fmin=45  InInit=[415, 0]  Ts=Ts
  Gain : Gain  Gain=1/sqrt(2)
  Gain2 : Gain  Gain=1/(415*sqrt(2)/sqrt(3))
  PLL (3ph) : spsPLL3phLib/PLL (3ph)  Fmin=45  Par_Init=[0, 50]  ParK=[180, 3200, 1]  TcD=1e-4  MaxRateChangeFreq=12  FilterCutOffFreq=25  Ts=Ts  AGC=on
  "Power (PLL-Driven, Positive-Sequence)" : spsPowerPLLDrivenPositiveSequenceLib/Power (PLL-Driven, Positive-Sequence)  Finit=50  Fmin=45  Vinit=[1, 0]  Iinit=[1, 0]  Ts=Ts
  Saturation1 : Saturate  UpperLimit=55  LowerLimit=45
  Terminator2 : Terminator
  Terminator4 : Terminator
  Freq : Outport
  P_kW : Outport  Port=2
  Q_kvar : Outport  Port=3
  Vab_rms : Outport  Port=4
  wires:
  Ipcc/1 -> "Power (PLL-Driven, Positive-Sequence)"/4
  Demux1/2 -> Add1/2
  PLL (3ph)/2 -> Fundamental (PLL-Driven)/2, "Power (PLL-Driven, Positive-Sequence)"/2
  PLL (3ph)/1 -> Saturation1/1
  Demux1/3 -> Terminator4/1
  Demux1/1 -> Add1/1
  Fundamental (PLL-Driven)/2 -> Terminator2/1
  Gain2/1 -> PLL (3ph)/1
  Vpcc/1 -> Demux1/1, "Power (PLL-Driven, Positive-Sequence)"/3, Gain2/1
  Add1/1 -> Fundamental (PLL-Driven)/3
  Fundamental (PLL-Driven)/1 -> Gain/1
  "Power (PLL-Driven, Positive-Sequence)"/1 -> P_kW/1
  "Power (PLL-Driven, Positive-Sequence)"/2 -> Q_kvar/1
  Saturation1/1 -> Freq/1, Fundamental (PLL-Driven)/1, "Power (PLL-Driven, Positive-Sequence)"/1
  Gain/1 -> Vab_rms/1

== system DFIG_and_Big_Generator/ Measurements1 ==
  Ipcc : Inport
  Vpcc : Inport  Port=2
  Add1 : Sum  Inputs=+-
  Demux1 : Demux  Outputs=3
  Fundamental (PLL-Driven) : spsFundamentalPLLDrivenLib/Fundamental (PLL-Driven)  Finit=50  Fmin=45  InInit=[415, 0]  Ts=Ts
  Gain : Gain  Gain=1/sqrt(2)
  Gain2 : Gain  Gain=1/(5000*sqrt(2)/sqrt(3))
  PLL (3ph) : spsPLL3phLib/PLL (3ph)  Fmin=45  Par_Init=[0, 50]  ParK=[180, 3200, 1]  TcD=1e-4  MaxRateChangeFreq=12  FilterCutOffFreq=25  Ts=Ts  AGC=on
  "Power (PLL-Driven, Positive-Sequence)" : spsPowerPLLDrivenPositiveSequenceLib/Power (PLL-Driven, Positive-Sequence)  Finit=50  Fmin=45  Vinit=[1, 0]  Iinit=[1, 0]  Ts=Ts
  Saturation1 : Saturate  UpperLimit=55  LowerLimit=45
  Terminator2 : Terminator
  Terminator4 : Terminator
  Freq : Outport
  P_kW : Outport  Port=2
  Q_kvar : Outport  Port=3
  Vab_rms : Outport  Port=4
  wires:
  Gain/1 -> Vab_rms/1
  Saturation1/1 -> "Power (PLL-Driven, Positive-Sequence)"/1, Fundamental (PLL-Driven)/1, Freq/1
  "Power (PLL-Driven, Positive-Sequence)"/2 -> Q_kvar/1
  "Power (PLL-Driven, Positive-Sequence)"/1 -> P_kW/1
  Fundamental (PLL-Driven)/1 -> Gain/1
  Add1/1 -> Fundamental (PLL-Driven)/3
  Vpcc/1 -> Gain2/1, "Power (PLL-Driven, Positive-Sequence)"/3, Demux1/1
  Gain2/1 -> PLL (3ph)/1
  Fundamental (PLL-Driven)/2 -> Terminator2/1
  Demux1/1 -> Add1/1
  Demux1/3 -> Terminator4/1
  PLL (3ph)/1 -> Saturation1/1
  PLL (3ph)/2 -> "Power (PLL-Driven, Positive-Sequence)"/2, Fundamental (PLL-Driven)/2
  Demux1/2 -> Add1/2
  Ipcc/1 -> "Power (PLL-Driven, Positive-Sequence)"/4

== system DFIG_and_Big_Generator/DC // AC Inverter ==
  note: Load
  Breaker : spsBreakerLib/Breaker  InitialState=1  SwitchingTimes=[11]  External=off  BreakerResistance=0.0001  SnubberResistance=1e6  SnubberCapacitance=inf  Measurements=None  MoreParameters=off  NoBreakLoop=off
  DC/AC Inverter : Subsystem
  Goto : Goto  TagVisibility=global
  Measure : spsThreePhaseVIMeasurementLib/Three-Phase V-I Measurement  VoltageMeasurement=phase-to-ground  SetLabelV=off  LabelV=V1  Vpu=on  VpuLL=off  CurrentMeasurement=no  SetLabelI=off  LabelI=I1  Ipu=off  Pbase=1e3  Vbase=4450  OutputType=Magnitude  PhasorSimulation=off  PSBequivalent=0
  Unit Delay1 : UnitDelay  SampleTime=Ts  HasFrameUpgradeWarning=on
  Voltage Regulator : Subsystem  mask(Voltage Regulator){Kp=0.8, Ki=100, Ts=Ts}
      mask prompts: Kp "Proportional gain  Kp:"; Ki "Integral gain Ki:"; Ts "Sample time (s) :"
  "Vref (pu) " : Constant
  Battery + : PMIOPort  Side=Left
  A : PMIOPort  Port=2  Side=Right
  B : PMIOPort  Port=3  Side=Right
  C : PMIOPort  Port=4  Side=Right
  Battery - : PMIOPort  Port=5  Side=Left
  wires:
  Unit Delay1/1 -> Goto/1
  "Vref (pu) "/1 -> Voltage Regulator/2(Vd_ref (pu))
  Measure/1 -> Voltage Regulator/1(Vabc (pu))
  Voltage Regulator/1(Vabc_inv) -> Unit Delay1/1
  connections:
  Measure/LConn1 -- DC/AC Inverter/RConn1
  Measure/LConn2 -- DC/AC Inverter/RConn2
  DC/AC Inverter/RConn3 -- Measure/LConn3
  A/RConn1 -- Measure/RConn1
  B/RConn1 -- Measure/RConn2
  C/RConn1 -- Measure/RConn3
  DC/AC Inverter/LConn2 -- Battery -/RConn1
  Breaker/LConn1 -- DC/AC Inverter/LConn1
  Breaker/RConn1 -- Battery +/RConn1
